simulink model "rosslerSystemLinearCurve"  (R2019a)
settings: Solver=ode4  StartTime=0  StopTime=10000  FixedStep=1e-3  RelTol=1e-3
settings Model: Creator=plazas  LastModifiedBy=Daples
settings DataIOCC: ReturnWorkspaceOutputs=off
settings OptimizationCC: DefaultParameterBehavior=Inlined
settings DebuggingCC: InitInArrayFormatMsg=none  ArithmeticOperatorsInVariantConditions=warning

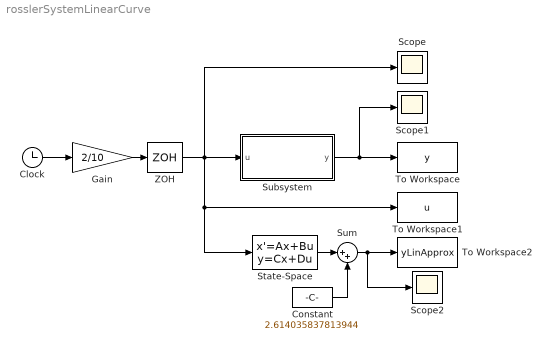
== system rosslerSystemLinearCurve ==
  Clock : Clock
  Constant : Constant  Value=2.614035837813944
      mask Display: disp('y0')
  Gain : Gain  Gain=2/10
  Scope : Scope
  Scope1 : Scope
  Scope2 : Scope
  State-Space : StateSpace  A=|  B=|  C=[0 0 1]  D=0  InitialCondition=[0 0 0]
      A=|
      | [0 -1.00000000000097 -1.00000000000097;
      | 1.00000000000321 0.200000000002409 0;
      | 2.61403583783170 0 -5.17717972249146]
      B=|
      | [0; 0;
      | 0.0133333333707242]
  Subsystem : Subsystem  mask{Ra=500, Rb=7500, Rc=17.5439, RCs=1, ci=[0.522807167562789; -2.614035837813944; 2.614035837813944]}
      mask prompts: Ra "Resistance a"; Rb "Resistance b"; Rc "Resistance c"; RCs "Time speed (RC)"; ci "Initial Conditions"
      mask init:
      | x10 = ci(1);
      | x20 = ci(2);
      | y0 = ci(3);
      mask Display: disp("Rössler Attractor")
  Sum : Sum  Inputs=|++
  To Workspace : ToWorkspace  VariableName=y  SampleTime=-1
  To Workspace1 : ToWorkspace  VariableName=u  SampleTime=-1
  To Workspace2 : ToWorkspace  VariableName=yLinApprox  SampleTime=-1
  "ZOH " : ZeroOrderHold  SampleTime=100
  wires:
  Clock/1 -> Gain/1
  Gain/1 -> "ZOH "/1
  Subsystem/1("y ") -> Scope1/1, To Workspace/1
  State-Space/1 -> Sum/1
  Constant/1 -> Sum/2
  Sum/1 -> Scope2/1, To Workspace2/1
  "ZOH "/1 -> State-Space/1, To Workspace1/1, Subsystem/1(u), Scope/1

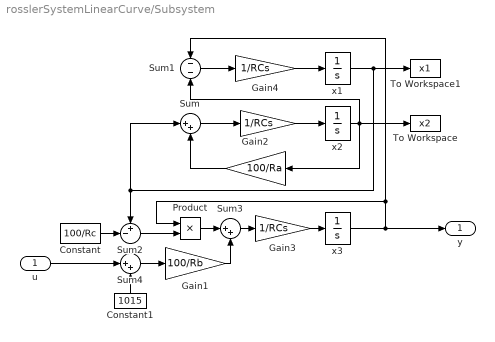
== system rosslerSystemLinearCurve/Subsystem ==
  u : Inport
  " " : Gain  Gain=1/RCs
  Constant : Constant  Value=100/Rc
  Constant1 : Constant  Value=1015
  Gain1 : Gain  Gain=100/Rb
  Gain2 : Gain  Gain=100/Ra
  Gain3 : Gain  Gain=1/RCs
  Gain4 : Gain  Gain=1/RCs
  Product : Product
  Sum : Sum  Inputs=|++
  Sum1 : Sum  Inputs=--
  Sum2 : Sum  Inputs=+-|
  Sum3 : Sum  Inputs=|++
  Sum4 : Sum  Inputs=|++
  To Workspace : ToWorkspace  VariableName=x2  SampleTime=-1
  To Workspace1 : ToWorkspace  VariableName=x1  SampleTime=-1
  x1 : Integrator  InitialCondition=x10
  x2 : Integrator  InitialCondition=x20
  "x3 " : Integrator  InitialCondition=y0
  "y " : Outport
  wires:
  Sum1/1 -> Gain4/1
  Gain2/1 -> Sum/2
  Sum2/1 -> Product/2
  Product/1 -> Sum3/1
  "x3 "/1 -> "y "/1, Sum1/1, Product/1
  x1/1 -> To Workspace1/1, Sum2/1, Sum/1
  Sum/1 -> " "/1
  Sum3/1 -> Gain3/1
  Constant/1 -> Sum2/2
  x2/1 -> Sum1/2, To Workspace/1, Gain2/1
  u/1 -> Sum4/1
  " "/1 -> x2/1
  Gain3/1 -> "x3 "/1
  Gain4/1 -> x1/1
  Gain1/1 -> Sum3/2
  Constant1/1 -> Sum4/2
  Sum4/1 -> Gain1/1
